simulink model "test"  (R2013b)
settings: Solver=ode45  StartTime=0.0  StopTime=70  RelTol=1e-3
libraries: xbsIndex_r4 x14, casper_library_misc x5, xps_library x1
settings Model: Creator=root  LastModifiedBy=root

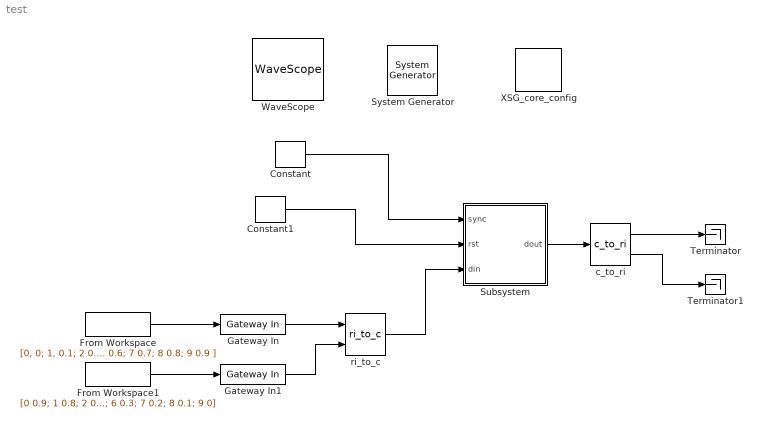
== system test ==
  " System Generator" : xbsIndex_r4/ System Generator  Tag=genX  xilinxfamily=Kintex7  part=xc7k325t  speed=-3  package=fbg676  synthesis_tool=XST  clock_wrapper=Clock Enables  directory=./netlist  proj_type=Project Navigator  Synth_file=XST Defaults  Impl_file=ISE Defaults  testbench=off  simulink_period=1  sysclk_period=10  dcm_input_clock_period=10  incr_netlist=off  trim_vbits=Everywhere in SubSystem  dbl_ovrd=According to Block Masks  core_generation=According to Block Masks  run_coregen=off  deprecated_control=off  eval_field=0  block_type=sysgen
  Constant : xbsIndex_r4/Constant  const=1  gui_display_data_type=Boolean  arith_type=Boolean  n_bits=16  bin_pt=14  preci_type=Single  exp_width=8  frac_width=24  explicit_period=on  period=1  equ=P=C  opselect=C  inp2=PCIN>>17  opr=+  inp1=P  carry=CIN  dbl_ovrd=off  block_type=constant
  Constant1 : xbsIndex_r4/Constant  const=0  gui_display_data_type=Boolean  arith_type=Boolean  n_bits=16  bin_pt=14  preci_type=Single  exp_width=8  frac_width=24  explicit_period=on  period=1  equ=P=C  opselect=C  inp2=PCIN>>17  opr=+  inp1=P  carry=CIN  dbl_ovrd=off  block_type=constant
  From Workspace : FromWorkspace  VariableName=[0, 0; 1, 0.1; 2 0.2; 3 0.3; 4 0.4; 5 0.5; 6 0.6; 7 0.7; 8 0.8; 9 0.9 ]  SampleTime=0  OutputAfterFinalValue=Holding final value
  From Workspace1 : FromWorkspace  VariableName=[0 0.9; 1 0.8; 2 0.7; 3 0.6; 4 0.5; 5 0.4; 6 0.3; 7 0.2; 8 0.1; 9 0]  SampleTime=0  OutputAfterFinalValue=Holding final value
  Gateway In : xbsIndex_r4/Gateway In  gui_display_data_type=Fixed-point  arith_type="Signed  (2's comp)"  n_bits=10  bin_pt=9  preci_type=Single  exp_width=8  frac_width=24  quantization="Round  (unbiased: +/- Inf)"  overflow=Saturate  period=1  dbl_ovrd=off  timing_constraint=None  locs_specified=off  LOCs={}  UseAsADC=off  ADCChannel='1'  inherit_from_input=off  hdl_port=on  block_type=gatewayin
  Gateway In1 : xbsIndex_r4/Gateway In  gui_display_data_type=Fixed-point  arith_type="Signed  (2's comp)"  n_bits=10  bin_pt=9  preci_type=Single  exp_width=8  frac_width=24  quantization="Round  (unbiased: +/- Inf)"  overflow=Saturate  period=1  dbl_ovrd=off  timing_constraint=None  locs_specified=off  LOCs={}  UseAsADC=off  ADCChannel='1'  inherit_from_input=off  hdl_port=on  block_type=gatewayin
  Subsystem : Subsystem  mask(msdft_comb){input_bitsize=10, fft_len=5, latency=0}
      mask prompts: fft_len "fft_len (2^?)"; latency "sub latency"
      mask init:
      | msdft_comb_init(gcb, ...
      |         'input_bitsize', input_bitsize, ...
      |         'fft_len', fft_len, ...
      |         'latency', latency);
      settings: AttributesFormatString=latency=0
  Terminator : Terminator
  Terminator1 : Terminator
  WaveScope : xbsIndex_r4/WaveScope  block_type=wavescope
  XSG_core_config : xps_library/XSG_core_config  Tag=xps:xsg  hw_sys=ROACH2:sx475t  clk_src=sys_clk  ROACH_clk_src=sys_clk  ROACH2_clk_src=sys_clk  MKDIG_clk_src=sys_clk  clk_rate=100  sample_period=1  synthesis_tool=XST
  c_to_ri : casper_library_misc/c_to_ri  n_bits=11  bin_pt=9
      settings: AttributesFormatString=11_9 r/i
  ri_to_c : casper_library_misc/ri_to_c
  wires:
  Constant/1 -> Subsystem/1(sync)
  Constant1/1 -> Subsystem/2(rst)
  Gateway In1/1 -> ri_to_c/2
  Gateway In/1 -> ri_to_c/1
  ri_to_c/1 -> Subsystem/3(din)
  Subsystem/1(dout) -> c_to_ri/1
  c_to_ri/1 -> Terminator/1
  c_to_ri/2 -> Terminator1/1
  From Workspace/1 -> Gateway In/1
  From Workspace1/1 -> Gateway In1/1

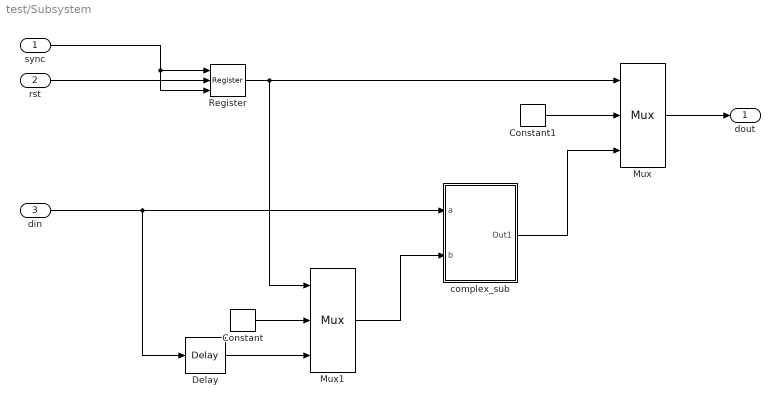
== system test/Subsystem ==
  sync : Inport
  rst : Inport  Port=2
  din : Inport  Port=3
  Constant : xbsIndex_r4/Constant  const=0  gui_display_data_type=Fixed-point  arith_type=Unsigned  n_bits=2*input_bitsize  bin_pt=0  preci_type=Single  exp_width=8  frac_width=24  explicit_period=on  period=1  equ=P=C  opselect=C  inp2=PCIN>>17  opr=+  inp1=P  carry=CIN  dbl_ovrd=off  block_type=constant
  Constant1 : xbsIndex_r4/Constant  const=0  gui_display_data_type=Fixed-point  arith_type=Unsigned  n_bits=2*(input_bitsize+1)  bin_pt=0  preci_type=Single  exp_width=8  frac_width=24  explicit_period=on  period=1  equ=P=C  opselect=C  inp2=PCIN>>17  opr=+  inp1=P  carry=CIN  dbl_ovrd=off  block_type=constant
  Delay : xbsIndex_r4/Delay  rst=off  infoeditControl=Selection of Reset will increase slice count due to use of real FFs and instead of SRLs  en=off  latency=2^fft_len  dbl_ovrd=off  reg_retiming=off  block_type=delay
  Mux : xbsIndex_r4/Mux  inputs=2  en=off  latency=0  precision=Full  arith_type=Unsigned  n_bits=16  bin_pt=14  quantization=Truncate  overflow=Wrap  dbl_ovrd=off  block_type=mux
  Mux1 : xbsIndex_r4/Mux  inputs=2  en=off  latency=0  precision=Full  arith_type=Unsigned  n_bits=16  bin_pt=14  quantization=Truncate  overflow=Wrap  dbl_ovrd=off  block_type=mux
  Register : xbsIndex_r4/Register  init=0  rst=on  en=on  dbl_ovrd=off  block_type=register
  complex_sub : Subsystem  mask(complex_sub){a_bitsize=input_bitsize, b_bitsize=input_bitsize, latency=0}
      mask init:
      | complex_sub_init(gcb, ...
      |             'a_bitsize', a_bitsize, ...
      |             'b_bitsize', b_bitsize, ...
      |             'latency', latency);
      settings: AttributesFormatString=latency=0
  dout : Outport
  wires:
  sync/1 -> Register/3, Register/1
  rst/1 -> Register/2
  Register/1 -> Mux1/1, Mux/1
  din/1 -> Delay/1, complex_sub/1("a ")
  complex_sub/1(Out1) -> Mux/3
  Delay/1 -> Mux1/3
  Constant/1 -> Mux1/2
  Constant1/1 -> Mux/2
  Mux1/1 -> complex_sub/2(b)
  Mux/1 -> dout/1

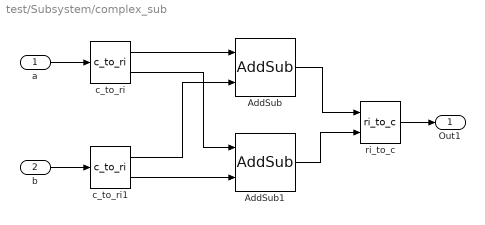
== system test/Subsystem/complex_sub ==
  "a " : Inport
  b : Inport  Port=2
  AddSub : xbsIndex_r4/AddSub  mode=Subtraction  use_carryin=off  use_carryout=off  en=off  latency=latency  precision=Full  arith_type=Unsigned  n_bits=16  bin_pt=14  quantization=Truncate  overflow=Wrap  dbl_ovrd=off  use_behavioral_HDL=off  hw_selection=Fabric  pipelined=off  block_type=addsub
  AddSub1 : xbsIndex_r4/AddSub  mode=Subtraction  use_carryin=off  use_carryout=off  en=off  latency=latency  precision=Full  arith_type=Unsigned  n_bits=16  bin_pt=14  quantization=Truncate  overflow=Wrap  dbl_ovrd=off  use_behavioral_HDL=off  hw_selection=Fabric  pipelined=off  block_type=addsub
  c_to_ri : casper_library_misc/c_to_ri  n_bits=a_bitsize  bin_pt=a_bitsize-1
      settings: AttributesFormatString=10_9 r/i
  c_to_ri1 : casper_library_misc/c_to_ri  n_bits=b_bitsize  bin_pt=b_bitsize-1
      settings: AttributesFormatString=10_9 r/i
  ri_to_c : casper_library_misc/ri_to_c
  Out1 : Outport
  wires:
  "a "/1 -> c_to_ri/1
  b/1 -> c_to_ri1/1
  c_to_ri/1 -> AddSub/1
  c_to_ri1/1 -> AddSub/2
  c_to_ri/2 -> AddSub1/1
  c_to_ri1/2 -> AddSub1/2
  AddSub/1 -> ri_to_c/1
  AddSub1/1 -> ri_to_c/2
  ri_to_c/1 -> Out1/1
